simulink model "FCS"  (R2019a)
settings: Solver=VariableStepAuto  StartTime=0.0  StopTime=10.0  RelTol=1e-3
undefined symbols (not defined in the file): argentina, ground, JD_0, Jw, namibia, nut80, r_ecef, t_orbit, v_ecef
libraries: dspmathops x12, vrlib x8, sc_toolbox x7
(part 1 of 2)
settings Model: Creator=mario  LastModifiedBy=mario
settings DataIOCC: ReturnWorkspaceOutputs=off
settings DebuggingCC: ArithmeticOperatorsInVariantConditions=warning
settings ModelReferenceCC: ModelReferenceNumInstancesAllowed=Single

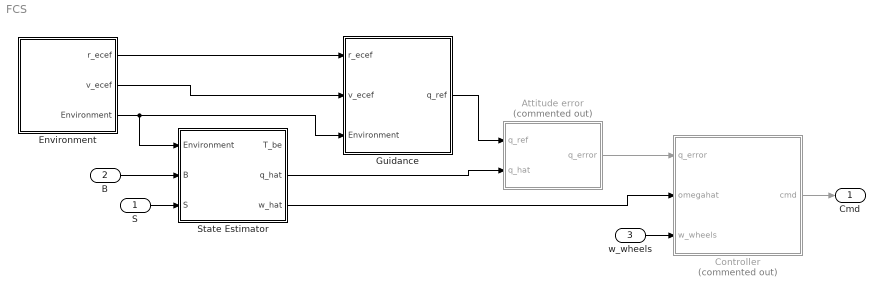
== system FCS ==
  S : Inport
  B : Inport  Port=2
  w_wheels : Inport  Port=3
  Attitude error : Subsystem  Commented=on
  Controller : Subsystem  Commented=on
  Environment : Subsystem
  Guidance : Subsystem
  State Estimator : Subsystem
  Cmd : Outport
  wires:
  Attitude error/1("q_error ") -> Controller/1(q_error)
  Controller/1(cmd) -> Cmd/1
  State Estimator/2(q_hat) -> Attitude error/2(q_hat)
  Guidance/1(q_ref) -> Attitude error/1(q_ref)
  w_wheels/1 -> Controller/3(w_wheels)
  State Estimator/3(w_hat) -> Controller/2(omegahat)
  B/1 -> State Estimator/2(B)
  S/1 -> State Estimator/3(S)
  Environment/1(r_ecef) -> Guidance/1(r_ecef)
  Environment/2(v_ecef) -> Guidance/2(v_ecef)
  Environment/3(Environment) -> State Estimator/1("Environment "), Guidance/3(Environment)

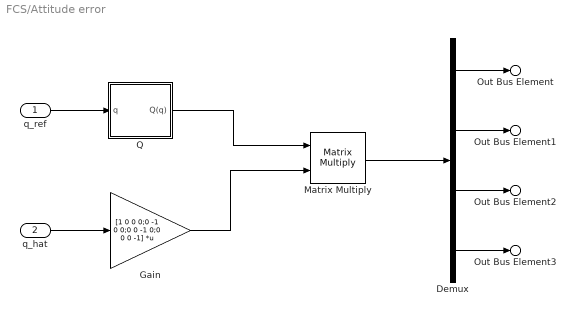
== system FCS/Attitude error ==
  q_ref : Inport
  q_hat : Inport  Port=2
  Demux : Demux
  Gain : Gain  Gain=[1 0 0 0;0 -1 0 0;0 0 -1 0;0 0 0 -1]  Multiplication=Matrix(K*u)
  Matrix Multiply : Product  Multiplication=Matrix(*)
  Q : Subsystem
  Out Bus Element : Outport  PortName=q_error  Element=q0
  Out Bus Element1 : Outport  PortName=q_error  Element=q1
  Out Bus Element2 : Outport  PortName=q_error  Element=q2
  Out Bus Element3 : Outport  PortName=q_error  Element=q3
  wires:
  q_ref/1 -> Q/1(q)
  q_hat/1 -> Gain/1
  Q/1(Q(q)) -> Matrix Multiply/1
  Gain/1 -> Matrix Multiply/2
  Matrix Multiply/1 -> Demux/1
  Demux/1 -> Out Bus Element/1
  Demux/3 -> Out Bus Element2/1
  Demux/2 -> Out Bus Element1/1
  Demux/4 -> Out Bus Element3/1

== system FCS/Controller ==
  q_error : Inport
  omegahat : Inport  Port=2
  w_wheels : Inport  Port=3
  Detumbling : Subsystem
  Momemtum unloading : Subsystem
  Three axis attitude controller : Subsystem
  cmd : Outport
  wires:
  Three axis attitude controller/1("cmd ") -> cmd/1
  q_error/1 -> Three axis attitude controller/1(q_error)
  omegahat/1 -> Three axis attitude controller/2(w_body)
  w_wheels/1 -> Momemtum unloading/1(w_wheels)

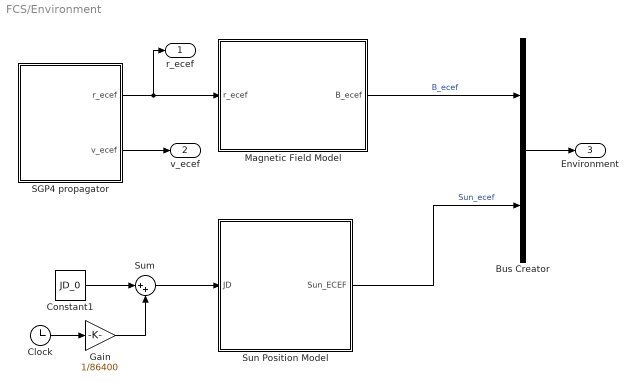
== system FCS/Environment ==
  Bus Creator : BusCreator  Inputs=2
  Clock : Clock
  Constant1 : Constant  Value=JD_0
  Gain : Gain  Gain=1/86400
  Magnetic Field Model : Subsystem
  SGP4 propagator : Subsystem
  Sum : Sum  Inputs=|++
  "Sun Position Model " : Subsystem
  r_ecef : Outport
  v_ecef : Outport  Port=2
  Environment : Outport  Port=3
  wires:
  Clock/1 -> Gain/1
  Constant1/1 -> Sum/1
  Gain/1 -> Sum/2
  Sum/1 -> "Sun Position Model "/1(JD)
  Magnetic Field Model/1(B_ecef) -> Bus Creator/1  "B_ecef"
  "Sun Position Model "/1(Sun_ECEF) -> Bus Creator/2  "Sun_ecef"
  Bus Creator/1 -> Environment/1
  SGP4 propagator/1(r_ecef) -> r_ecef/1, Magnetic Field Model/1(r_ecef)
  SGP4 propagator/2(v_ecef) -> v_ecef/1

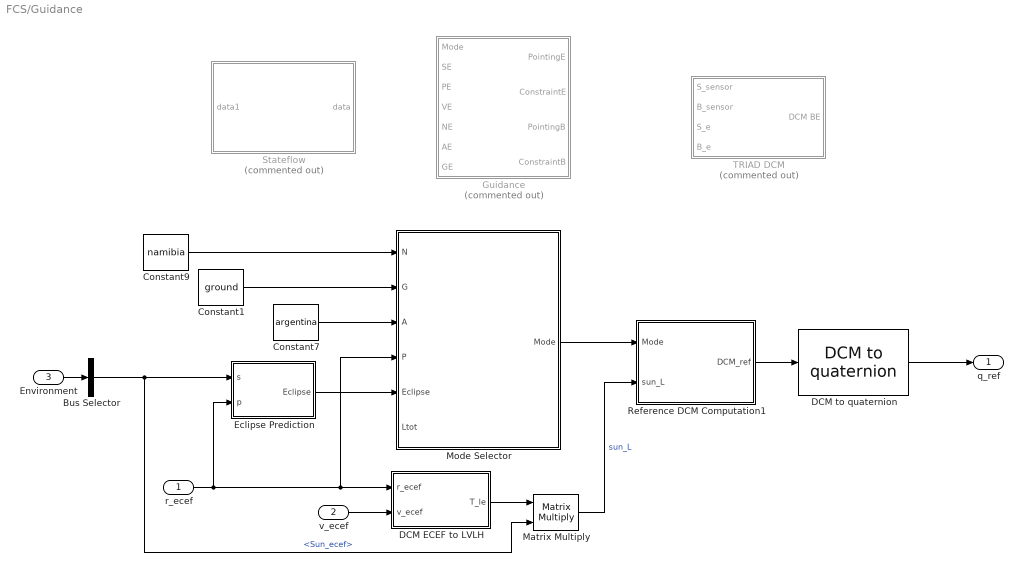
== system FCS/Guidance ==
  r_ecef : Inport
  v_ecef : Inport  Port=2
  Environment : Inport  Port=3
  Bus Selector : BusSelector  OutputSignals=Sun_ecef
  Constant1 : Constant  Value=ground
  Constant7 : Constant  Value=argentina
  Constant9 : Constant  Value=namibia
  DCM ECEF to LVLH : Subsystem
  DCM to quaternion : sc_toolbox/Kinematics/DCM to quaternion  SystemSampleTime=-1
      settings: SourceProductName=Spacecraft Toolbox
  Eclipse Prediction : MATLAB Function  TreatAsAtomicUnit=on
  Guidance : MATLAB Function  Commented=on  TreatAsAtomicUnit=on
  Matrix Multiply : Product  Multiplication=Matrix(*)
  Mode Selector : MATLAB Function  TreatAsAtomicUnit=on
  Reference DCM Computation1 : MATLAB Function  TreatAsAtomicUnit=on
  Stateflow : Stateflow chart  Commented=on  TreatAsAtomicUnit=on
  TRIAD DCM : Subsystem  Commented=on
  q_ref : Outport  VectorParamsAs1DForOutWhenUnconnected=on
  wires:
  Constant1/1 -> Mode Selector/2(G)
  Constant9/1 -> Mode Selector/1(N)
  Constant7/1 -> Mode Selector/3(A)
  Eclipse Prediction/1(Eclipse) -> Mode Selector/5(Eclipse)
  Mode Selector/1(Mode) -> Reference DCM Computation1/1(Mode)
  v_ecef/1 -> DCM ECEF to LVLH/2(v_ecef)
  DCM to quaternion/1 -> q_ref/1
  Reference DCM Computation1/1(DCM_ref) -> DCM to quaternion/1
  r_ecef/1 -> Eclipse Prediction/2(p), DCM ECEF to LVLH/1(r_ecef), Mode Selector/4(P)
  Environment/1 -> Bus Selector/1
  Bus Selector/1 -> Matrix Multiply/2, Eclipse Prediction/1(s)  "<Sun_ecef>"
  DCM ECEF to LVLH/1(T_le) -> Matrix Multiply/1
  Matrix Multiply/1 -> Reference DCM Computation1/2(sun_L)  "sun_L"

== system FCS/State Estimator ==
  "Environment " : Inport
  B : Inport  Port=2
  S : Inport  Port=3
  Bus Selector : BusSelector  OutputSignals=B_ecef,Sun_ecef
  Extended Kalman Filter : MATLAB Function  Commented=on  TreatAsAtomicUnit=on
  TRIAD DCM : Subsystem
  T_be : Outport
  q_hat : Outport  Port=2
  w_hat : Outport  Port=3
  wires:
  B/1 -> TRIAD DCM/2(B_sensor), Extended Kalman Filter/1(B)
  S/1 -> TRIAD DCM/1(S_sensor), Extended Kalman Filter/2(S)
  Extended Kalman Filter/2(what) -> w_hat/1
  Extended Kalman Filter/1(qhat) -> q_hat/1
  TRIAD DCM/1(DCM BE) -> T_be/1
  "Environment "/1 -> Bus Selector/1
  Bus Selector/1 -> TRIAD DCM/3(B_e)  "<B_ecef>"
  Bus Selector/2 -> TRIAD DCM/4(S_e)  "<Sun_ecef>"

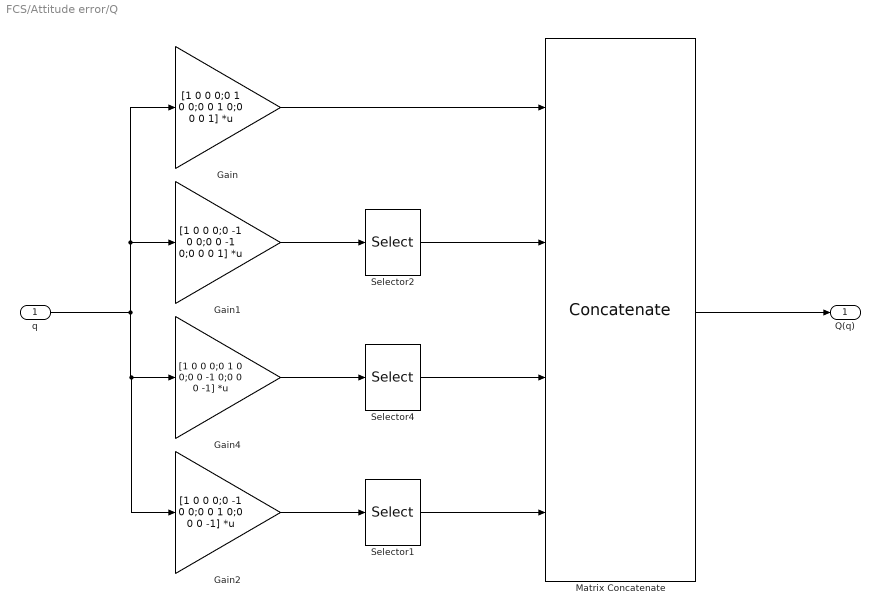
== system FCS/Attitude error/Q ==
  q : Inport
  Gain : Gain  Gain=[1 0 0 0;0 1 0 0;0 0 1 0;0 0 0 1]  Multiplication=Matrix(K*u)
  Gain1 : Gain  Gain=[1 0 0 0;0 -1 0 0;0 0 -1 0;0 0 0 1]  Multiplication=Matrix(K*u)
  Gain2 : Gain  Gain=[1 0 0 0;0 -1 0 0;0 0 1 0;0 0 0 -1]  Multiplication=Matrix(K*u)
  Gain4 : Gain  Gain=[1 0 0 0;0 1 0 0;0 0 -1 0;0 0 0 -1]  Multiplication=Matrix(K*u)
  Matrix Concatenate : Concatenate  NumInputs=4  Mode=Multidimensional array  ConcatenateDimension=2
  Selector1 : Selector  InputPortWidth=4  IndexOptions=Index vector (dialog)  Indices=[4 3 2 1]  OutputSizes=1
  Selector2 : Selector  InputPortWidth=4  IndexOptions=Index vector (dialog)  Indices=[2 1 4 3]  OutputSizes=1
  Selector4 : Selector  InputPortWidth=4  IndexOptions=Index vector (dialog)  Indices=[3 4 1 2]  OutputSizes=1
  Q(q) : Outport
  wires:
  Gain1/1 -> Selector2/1
  Gain/1 -> Matrix Concatenate/1
  q/1 -> Gain2/1, Gain4/1, Gain1/1, Gain/1
  Selector4/1 -> Matrix Concatenate/3
  Matrix Concatenate/1 -> Q(q)/1
  Selector2/1 -> Matrix Concatenate/2
  Gain4/1 -> Selector4/1
  Gain2/1 -> Selector1/1
  Selector1/1 -> Matrix Concatenate/4

== system FCS/Controller/Detumbling ==
  In1 : Inport
  cmd : Outport
  wires:
  In1/1 -> cmd/1

== system FCS/Controller/Momemtum unloading ==
  w_wheels : Inport
  cmd : Outport
  wires:
  w_wheels/1 -> cmd/1

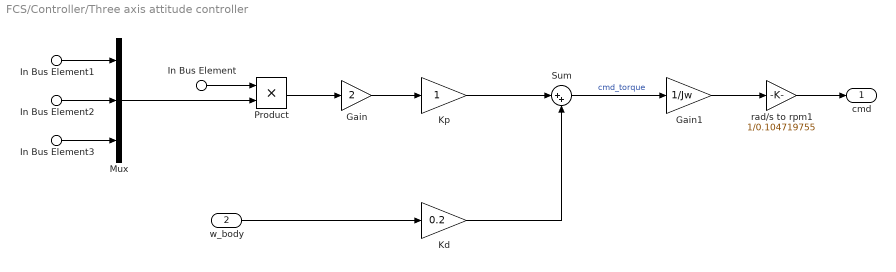
== system FCS/Controller/Three axis attitude controller ==
  In Bus Element : Inport  PortName=q_error  Element=q0
  In Bus Element1 : Inport  PortName=q_error  Element=q1
  In Bus Element2 : Inport  PortName=q_error  Element=q2
  In Bus Element3 : Inport  PortName=q_error  Element=q3
  w_body : Inport  Port=2
  Gain : Gain  Gain=2
  Gain1 : Gain  Gain=1/Jw
  Kd : Gain  Gain=0.2
  Kp : Gain
  Mux : Mux  Inputs=3
  Product : Product
  Sum : Sum  Inputs=|++
  rad/s to rpm1 : Gain  Gain=1/0.104719755
  "cmd " : Outport
  wires:
  w_body/1 -> Kd/1
  In Bus Element1/1 -> Mux/1
  Gain1/1 -> rad/s to rpm1/1
  Mux/1 -> Product/2
  Gain/1 -> Kp/1
  Product/1 -> Gain/1
  Kd/1 -> Sum/2
  In Bus Element2/1 -> Mux/2
  rad/s to rpm1/1 -> "cmd "/1
  In Bus Element/1 -> Product/1
  In Bus Element3/1 -> Mux/3
  Sum/1 -> Gain1/1  "cmd_torque"
  Kp/1 -> Sum/1

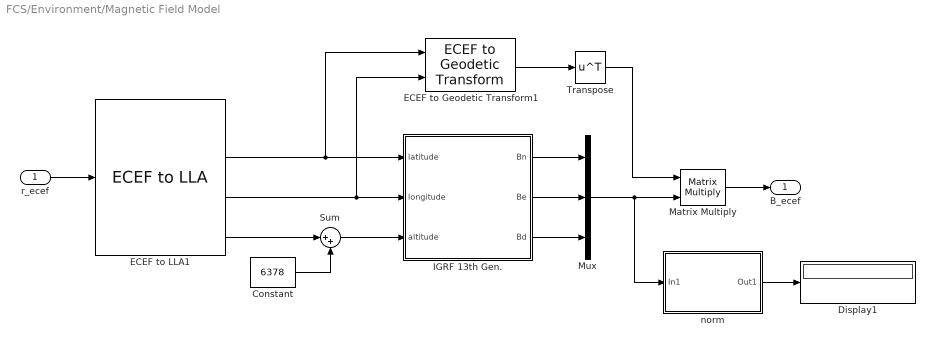
== system FCS/Environment/Magnetic Field Model ==
  r_ecef : Inport
  Constant : Constant  Value=6378
  Display1 : Display
  ECEF to Geodetic Transform1 : sc_toolbox/Coordinates Transformations/ECEF to Geodetic Transform  SystemSampleTime=-1
      settings: SourceProductName=Spacecraft Toolbox
  ECEF to LLA1 : sc_toolbox/Coordinates Transformations/ECEF to LLA  SystemSampleTime=-1
      settings: SourceProductName=Spacecraft Toolbox
  IGRF 13th Gen. : MATLAB Function  TreatAsAtomicUnit=on
  Matrix Multiply : Product  Multiplication=Matrix(*)
  Mux : Mux  Inputs=3
  Sum : Sum  Inputs=|++
  Transpose : Math  Operator=transpose  SaturateOnIntegerOverflow=on
  norm : Subsystem
  B_ecef : Outport  VectorParamsAs1DForOutWhenUnconnected=on
  wires:
  IGRF 13th Gen./2(Be) -> Mux/2
  IGRF 13th Gen./3(Bd) -> Mux/3
  IGRF 13th Gen./1(Bn) -> Mux/1
  r_ecef/1 -> ECEF to LLA1/1
  ECEF to LLA1/3 -> ECEF to Geodetic Transform1/2, IGRF 13th Gen./2(longitude)
  ECEF to LLA1/2 -> ECEF to Geodetic Transform1/1, IGRF 13th Gen./1(latitude)
  ECEF to LLA1/4 -> Sum/1
  Mux/1 -> Matrix Multiply/2, norm/1(In1)
  Sum/1 -> IGRF 13th Gen./3(altitude)
  Constant/1 -> Sum/2
  norm/1(Out1) -> Display1/1
  ECEF to Geodetic Transform1/1 -> Transpose/1
  Matrix Multiply/1 -> B_ecef/1
  Transpose/1 -> Matrix Multiply/1

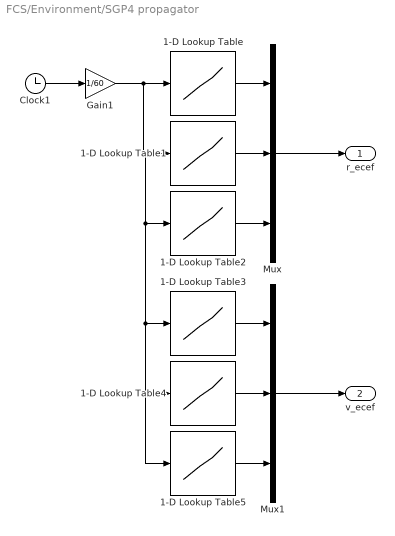
== system FCS/Environment/SGP4 propagator ==
  1-D Lookup Table : Lookup_n-D  NumberOfTableDimensions=1  BreakpointsForDimension1=t_orbit  BreakpointsForDimension2=t_orbit  BreakpointsForDimension3=t_orbit  Table=r_ecef(:,1)  InternalRulePriority=Speed  RndMeth=Simplest  InputSameDT=on
  1-D Lookup Table1 : Lookup_n-D  NumberOfTableDimensions=1  BreakpointsForDimension1=t_orbit  BreakpointsForDimension2=t_orbit  BreakpointsForDimension3=t_orbit  Table=r_ecef(:,2)  InternalRulePriority=Speed  RndMeth=Simplest  InputSameDT=on
  1-D Lookup Table2 : Lookup_n-D  NumberOfTableDimensions=1  BreakpointsForDimension1=t_orbit  BreakpointsForDimension2=t_orbit  BreakpointsForDimension3=t_orbit  Table=r_ecef(:,3)  InternalRulePriority=Speed  RndMeth=Simplest  InputSameDT=on
  1-D Lookup Table3 : Lookup_n-D  NumberOfTableDimensions=1  BreakpointsForDimension1=t_orbit  BreakpointsForDimension2=t_orbit  BreakpointsForDimension3=t_orbit  Table=v_ecef(:,1)  InternalRulePriority=Speed  RndMeth=Simplest  InputSameDT=on
  1-D Lookup Table4 : Lookup_n-D  NumberOfTableDimensions=1  BreakpointsForDimension1=t_orbit  BreakpointsForDimension2=t_orbit  BreakpointsForDimension3=t_orbit  Table=v_ecef(:,2)  InternalRulePriority=Speed  RndMeth=Simplest  InputSameDT=on
  1-D Lookup Table5 : Lookup_n-D  NumberOfTableDimensions=1  BreakpointsForDimension1=t_orbit  BreakpointsForDimension2=t_orbit  BreakpointsForDimension3=t_orbit  Table=v_ecef(:,3)  InternalRulePriority=Speed  RndMeth=Simplest  InputSameDT=on
  Clock1 : Clock
  Gain1 : Gain  Gain=1/60
  Mux : Mux  Inputs=3
  Mux1 : Mux  Inputs=3
  r_ecef : Outport  VectorParamsAs1DForOutWhenUnconnected=on
  v_ecef : Outport  Port=2
  wires:
  1-D Lookup Table2/1 -> Mux/3
  Gain1/1 -> 1-D Lookup Table5/1, 1-D Lookup Table4/1, 1-D Lookup Table3/1, 1-D Lookup Table2/1, 1-D Lookup Table1/1, 1-D Lookup Table/1
  Clock1/1 -> Gain1/1
  1-D Lookup Table1/1 -> Mux/2
  1-D Lookup Table/1 -> Mux/1
  Mux/1 -> r_ecef/1
  1-D Lookup Table3/1 -> Mux1/1
  1-D Lookup Table4/1 -> Mux1/2
  1-D Lookup Table5/1 -> Mux1/3
  Mux1/1 -> v_ecef/1

== system FCS/Environment/Sun Position Model  ==
  JD : Inport
  MOD to ECEF : Subsystem
  Sun Position Vector : MATLAB Function  TreatAsAtomicUnit=on
  Sun_ECEF : Outport
  wires:
  Sun Position Vector/1(rsun) -> MOD to ECEF/1(Sun_MOD)
  JD/1 -> MOD to ECEF/2(JD), Sun Position Vector/1(jd)
  MOD to ECEF/1(Sun_ECEF) -> Sun_ECEF/1

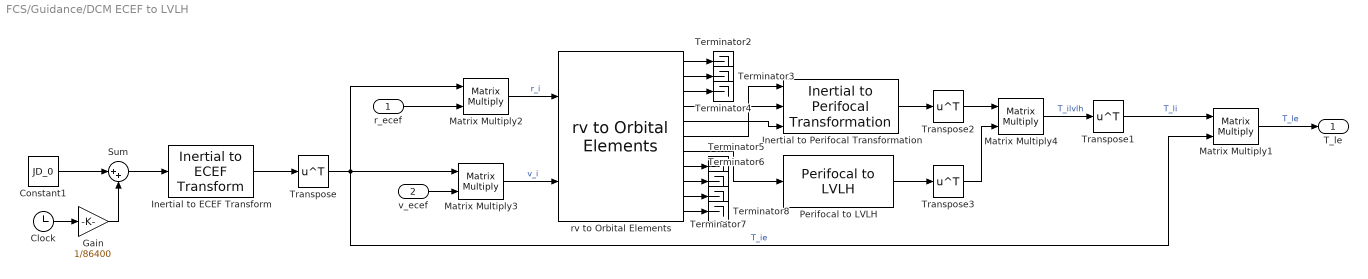
== system FCS/Guidance/DCM ECEF to LVLH ==
  r_ecef : Inport
  v_ecef : Inport  Port=2
  Clock : Clock
  Constant1 : Constant  Value=JD_0
  Gain : Gain  Gain=1/86400
  Inertial to ECEF Transform : sc_toolbox/Inertial to ECEF Transform  SystemSampleTime=-1
      settings: SourceProductName=Spacecraft Toolbox
  Inertial to Perifocal Transformation : sc_toolbox/Inertial to Perifocal Transformation  SystemSampleTime=-1
      settings: SourceProductName=Spacecraft Toolbox
  Matrix Multiply{1..4} (4 alike) : Product  Multiplication=Matrix(*)
  Perifocal to LVLH : sc_toolbox/Perifocal to LVLH  SystemSampleTime=-1
      settings: SourceProductName=Spacecraft Toolbox
  Sum : Sum  Inputs=|++
  Terminator{2..8} (7 alike) : Terminator
  Transpose{,1..3} (4 alike) : Math  Operator=transpose  SaturateOnIntegerOverflow=on
  rv to Orbital Elements : sc_toolbox/rv to Orbital Elements  SystemSampleTime=-1
      settings: SourceProductName=Spacecraft Toolbox
  T_le : Outport
  wires:
  rv to Orbital Elements/7 -> Perifocal to LVLH/1
  Matrix Multiply4/1 -> Transpose1/1  "T_ilvlh"
  Transpose3/1 -> Matrix Multiply4/2
  Matrix Multiply2/1 -> rv to Orbital Elements/1  "r_i"
  rv to Orbital Elements/2 -> Terminator3/1
  Perifocal to LVLH/1 -> Transpose3/1
  Transpose2/1 -> Matrix Multiply4/1
  rv to Orbital Elements/1 -> Terminator2/1
  rv to Orbital Elements/8 -> Terminator5/1
  rv to Orbital Elements/3 -> Terminator4/1
  Inertial to Perifocal Transformation/1 -> Transpose2/1
  rv to Orbital Elements/6 -> Inertial to Perifocal Transformation/1
  rv to Orbital Elements/11 -> Terminator8/1
  Matrix Multiply3/1 -> rv to Orbital Elements/2  "v_i"
  rv to Orbital Elements/5 -> Inertial to Perifocal Transformation/3
  rv to Orbital Elements/10 -> Terminator7/1
  rv to Orbital Elements/9 -> Terminator6/1
  rv to Orbital Elements/4 -> Inertial to Perifocal Transformation/2
  v_ecef/1 -> Matrix Multiply3/2
  Sum/1 -> Inertial to ECEF Transform/1
  Inertial to ECEF Transform/1 -> Transpose/1
  Constant1/1 -> Sum/1
  Gain/1 -> Sum/2
  Clock/1 -> Gain/1
  r_ecef/1 -> Matrix Multiply2/2
  Matrix Multiply1/1 -> T_le/1  "T_le"
  Transpose1/1 -> Matrix Multiply1/1  "T_li"
  Transpose/1 -> Matrix Multiply1/2, Matrix Multiply2/1, Matrix Multiply3/1  "T_ie"

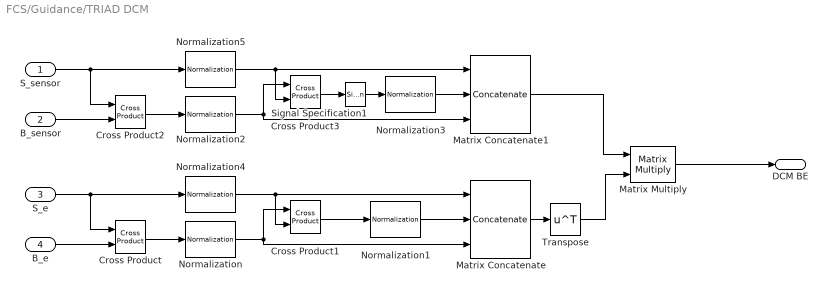
== system FCS/Guidance/TRIAD DCM ==
  S_sensor : Inport
  B_sensor : Inport  Port=2
  S_e : Inport  Port=3
  B_e : Inport  Port=4
  Cross Product{,1..3} (4 alike) : vrlib/Utilities/Cross Product
      settings: SourceProductBaseCode=VR
  Matrix Concatenate : Concatenate  NumInputs=3  Mode=Multidimensional array  ConcatenateDimension=2
  Matrix Concatenate1 : Concatenate  NumInputs=3  Mode=Multidimensional array  ConcatenateDimension=2
  Matrix Multiply : Product  Multiplication=Matrix(*)
  Normalization{,1..5} (6 alike) : dspmathops/Normalization  NormType=2-norm  Bias=1e-10  NormOver=Each column  Dimension=1  roundingMode=Floor  overflowMode=off  accumDataTypeStr=Inherit: Same as product output  accumLastDataTypeStr=Inherit: Same as product output  outputDataTypeStr=Inherit: Same as product output  outputMin=[]  outputMax=[]  outputLastDataTypeStr=Inherit: Same as product output
      settings: SourceProductName=DSP System Toolbox
  Signal Specification1 : SignalSpecification  Dimensions=3
  Transpose : Math  Operator=transpose  SaturateOnIntegerOverflow=on
  DCM BE : Outport
  wires:
  Normalization/1 -> Matrix Concatenate/3, Cross Product1/1
  Normalization5/1 -> Matrix Concatenate1/1, Cross Product3/2
  Cross Product1/1 -> Normalization1/1
  Normalization3/1 -> Matrix Concatenate1/2
  Cross Product3/1 -> Signal Specification1/1
  B_e/1 -> Cross Product/2
  Normalization4/1 -> Matrix Concatenate/1, Cross Product1/2
  S_e/1 -> Normalization4/1, Cross Product/1
  Cross Product2/1 -> Normalization2/1
  Cross Product/1 -> Normalization/1
  Normalization1/1 -> Matrix Concatenate/2
  Normalization2/1 -> Cross Product3/1, Matrix Concatenate1/3
  Matrix Concatenate/1 -> Transpose/1
  Matrix Concatenate1/1 -> Matrix Multiply/1
  Transpose/1 -> Matrix Multiply/2
  S_sensor/1 -> Cross Product2/1, Normalization5/1
  B_sensor/1 -> Cross Product2/2
  Matrix Multiply/1 -> DCM BE/1
  Signal Specification1/1 -> Normalization3/1

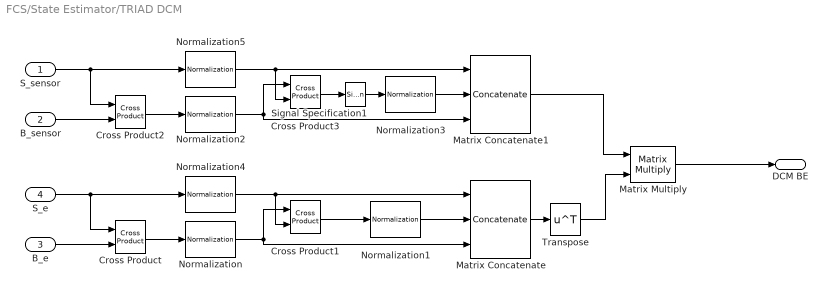
== system FCS/State Estimator/TRIAD DCM ==
  S_sensor : Inport
  B_sensor : Inport  Port=2
  B_e : Inport  Port=3
  S_e : Inport  Port=4
  Cross Product{,1..3} (4 alike) : vrlib/Utilities/Cross Product
      settings: SourceProductBaseCode=VR
  Matrix Concatenate : Concatenate  NumInputs=3  Mode=Multidimensional array  ConcatenateDimension=2
  Matrix Concatenate1 : Concatenate  NumInputs=3  Mode=Multidimensional array  ConcatenateDimension=2
  Matrix Multiply : Product  Multiplication=Matrix(*)
  Normalization{,1..5} (6 alike) : dspmathops/Normalization  NormType=2-norm  Bias=1e-10  NormOver=Each column  Dimension=1  roundingMode=Floor  overflowMode=off  accumDataTypeStr=Inherit: Same as product output  accumLastDataTypeStr=Inherit: Same as product output  outputDataTypeStr=Inherit: Same as product output  outputMin=[]  outputMax=[]  outputLastDataTypeStr=Inherit: Same as product output
      settings: SourceProductName=DSP System Toolbox
  Signal Specification1 : SignalSpecification  Dimensions=3
  Transpose : Math  Operator=transpose  SaturateOnIntegerOverflow=on
  DCM BE : Outport
  wires:
  Normalization/1 -> Matrix Concatenate/3, Cross Product1/1
  Normalization5/1 -> Matrix Concatenate1/1, Cross Product3/2
  Cross Product1/1 -> Normalization1/1
  Normalization3/1 -> Matrix Concatenate1/2
  Cross Product3/1 -> Signal Specification1/1
  B_e/1 -> Cross Product/2
  Normalization4/1 -> Matrix Concatenate/1, Cross Product1/2
  S_e/1 -> Normalization4/1, Cross Product/1
  Cross Product2/1 -> Normalization2/1
  Cross Product/1 -> Normalization/1
  Normalization1/1 -> Matrix Concatenate/2
  Normalization2/1 -> Cross Product3/1, Matrix Concatenate1/3
  Matrix Concatenate/1 -> Transpose/1
  Matrix Concatenate1/1 -> Matrix Multiply/1
  Transpose/1 -> Matrix Multiply/2
  S_sensor/1 -> Cross Product2/1, Normalization5/1
  B_sensor/1 -> Cross Product2/2
  Matrix Multiply/1 -> DCM BE/1
  Signal Specification1/1 -> Normalization3/1

== system FCS/Environment/Magnetic Field Model/norm ==
  In1 : Inport
  Add : Sum  Inputs=+++
  Demux : Demux  Outputs=3
  Product : Product
  Product1 : Product
  Product2 : Product
  Sqrt : Sqrt  SaturateOnIntegerOverflow=on
  Out1 : Outport
  wires:
  Demux/2 -> Product1/2, Product1/1
  Demux/1 -> Product/2, Product/1
  Sqrt/1 -> Out1/1
  Product2/1 -> Add/3
  Product1/1 -> Add/2
  Product/1 -> Add/1
  Add/1 -> Sqrt/1
  Demux/3 -> Product2/2, Product2/1
  In1/1 -> Demux/1

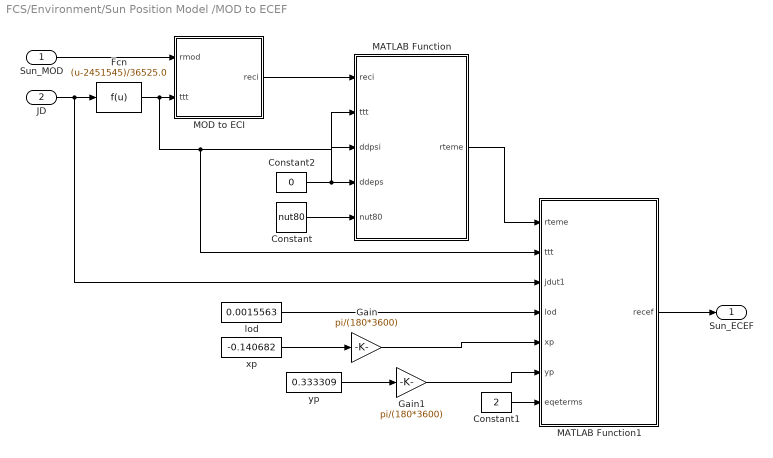
== system FCS/Environment/Sun Position Model /MOD to ECEF ==
  Sun_MOD : Inport
  JD : Inport  Port=2
  Constant : Constant  Value=nut80
  Constant1 : Constant  Value=2
  Constant2 : Constant  Value=0
  Fcn : Fcn  Expr=(u-2451545)/36525.0
  Gain : Gain  Gain=pi/(180*3600)
  Gain1 : Gain  Gain=pi/(180*3600)
  MATLAB Function : MATLAB Function  TreatAsAtomicUnit=on
  MATLAB Function1 : MATLAB Function  TreatAsAtomicUnit=on
  MOD to ECI : MATLAB Function  TreatAsAtomicUnit=on
  lod : Constant  Value=0.0015563
  xp : Constant  Value=-0.140682
  yp : Constant  Value=0.333309
  Sun_ECEF : Outport
  wires:
  Sun_MOD/1 -> MOD to ECI/1(rmod)
  Fcn/1 -> MATLAB Function1/2(ttt), MATLAB Function/2(ttt), MOD to ECI/2(ttt)
  JD/1 -> MATLAB Function1/3(jdut1), Fcn/1
  MOD to ECI/1(reci) -> MATLAB Function/1(reci)
  Constant2/1 -> MATLAB Function/4(ddeps), MATLAB Function/3(ddpsi)
  MATLAB Function1/1(recef) -> Sun_ECEF/1
  MATLAB Function/1(rteme) -> MATLAB Function1/1(rteme)
  Constant/1 -> MATLAB Function/5(nut80)
  Constant1/1 -> MATLAB Function1/7(eqeterms)
  lod/1 -> MATLAB Function1/4(lod)
  Gain/1 -> MATLAB Function1/5(xp)
  yp/1 -> Gain1/1
  xp/1 -> Gain/1
  Gain1/1 -> MATLAB Function1/6(yp)

== matlab function FCS/State Estimator/Extended Kalman Filter ==
  data: B input; qhat output; S input; what output
function [qhat,what] = ekf(B,S)
% QUATERNIONS EKF

% Initialization
T = 1/30;
g = 9.81;
n = length(acc);
euler = zeros(n,3);
euler(1,:) = [0 0 0];

x_hatp = [euler3212q(euler(1,:));zeros(3,1)];
Pp = 0.0001*eye(7);
R =diag([8e-4;8e-4;8e-4]);
qq = 0.0001;
qb = 1e-5;
Q =diag([qq;qq;qq;qq;qb;qb;qb]);

for i = 1:n
    
    Sq = [-x_hatp(2) -x_hatp(3) -x_hatp(4);
    x_hatp(1) -x_hatp(4) x_hatp(3);
    x_hatp(4) x_hatp(1) -x_hatp(2);
    -x_hatp(3) x_hatp(2) x_hatp(1)];

    Sw = [0 -gyr(i,1) -gyr(i,2) -gyr(i,3);
        gyr(i,1) 0 gyr(i,3) -gyr(i,2);
        gyr(i,2) -gyr(i,3) 0 gyr(i,1);
        gyr(i,3) gyr(i,2) -gyr(i,1) 0]; 
    
    F = [0.5*Sw -0.5*Sq;
        zeros(3,4) zeros(3,3)];
    
    Phi = expm(F*T);
    func = @(x)Phi*Q*Phi';
    Q_m = integral(func,0,T,'ArrayValued',1,'RelTol',5);
    
    Qk = [T^3/12*(qq*(eye(4)+Sw)*(eye(4)+Sw'))+qb*Sq*(Sq') -T^2/4*qb*Sq;
        -T^2/4*qb*Sq' T*qb*eye(3)];
    
    % Propagation

    x_hatm = Phi*x_hatp;
    Pm = Phi*Pp*Phi' + Q_m;
    %x_hatm(1:4) = x_hatm(1:4)/norm(x_hatm(1:4));
    
    % Measurement

    H =  2*[-x_hatm(3) x_hatm(4) -x_hatm(1) x_hatm(2) zeros(1,3);
                x_hatm(2) x_hatm(1) x_hatm(4) x_hatm(3) zeros(1,3);
                x_hatm(1) -x_hatm(2) -x_hatm(3) x_hatm(4) zeros(1,3)];

    y_hat = H*x_hatm;
    S = (H*Pm*H'+R);
    K = (H*Pm)'/S;

    % Update
    y = [acc(i,1)/g acc(i,2)/g acc(i,3)/g]';
    x_hatp = x_hatm + K*(y - y_hat);
    Pp = (eye(7) - K*H)*Pm;
    
    x_hatp(1:4) = x_hatp(1:4)/norm(x_hatp(1:4));
    euler(i,:) = q2euler(x_hatp(1:4));
    
end

== stateflow chart FCS/Guidance/Stateflow ==
  state Mission_modes
    state Idle
    state Imaging
    (default) -> Idle
  (default) -> Mission_modes
  data: data output; data1 input

== matlab function FCS/Environment/Magnetic Field Model/IGRF 13th Gen. ==
  data: latitude input; Bn output; longitude input; altitude input; Be output; Bd output
function [Bn, Be, Bd] = igrf(latitude, longitude, altitude)

%REMOVED COORD AS EVERYTHING IS ALREADY IN GEOCENTRIC. KEEPING TIME FOR NOW

% IGRF Earth's magnetic field from IGRF model.
% 
% Usage: [BX, BY, BZ] = IGRF(TIME, LATITUDE, LONGITUDE, ALTITUDE, COORD)
%     or [BX, BY, BZ] = IGRF(COEFS, LATITUDE, LONGITUDE, ALTITUDE, COORD)
%     or B = IGRF(TIME, LATITUDE, LONGITUDE, ALTITUDE, COORD)
%     or B = IGRF(COEFS, LATITUDE, LONGITUDE, ALTITUDE, COORD)
% 
% Calculates the components of the Earth's magnetic field using the
% International Geomagnetic Reference Field (IGRF) model. The inputs for
% the position can be scalars or vectors (in the latter case each should
% have the same number of elements or be a scalar), but TIME must be a
% scalar.
% 
% When all the coordinate inputs are scalars, the function can be run more
% efficiently by providing the proper IGRF coefficient vector for a given
% time rather than the time itself. This mode is useful when making
% multiple calls to the function while keeping the time the same (meaning
% the coefficients will be the same for each run) as loading the
% coefficients can be the most time-consuming part of the function. The
% coefficient vector can be easily loaded using the function LOADIGRFCOEFS.
% This mode is assumed when all the coordinate inputs are scalars and the
% first input is a vector. In this case, the coefficient vector should be
% formatted as (LOADIGRFCOEFS provides this):
% 
%   [g(n=1,m=0) g(n=1,m=1) h(n=1,m=1) g(n=2,m=0) g(n=2,m=1) h(n=2,m=1) ...]
% 
% Regardless of the size of the inputs, the outputs will be column vectors.
% If only one output is requested, B = [BX(:), BY(:), BZ(:)] is output.
% Note that the other parameters the IGRF gives can be computed from BX,
% BY, and BZ as:
% 
%   Horizonal intensity: hypot(BX, BY) (i.e., sqrt(BX.^2 + BY.^2) )
%   Total intensity: hypot(BX, hypot(BY, BZ))
%   Declination: atan2(BY, BX)
%   Inclination: atan(BZ./hypot(BX, BY))
% 
% This function relies on having the file igrfcoefs.mat in the MATLAB
% path to function properly when a time is input. If this file cannot be
% found, this function will try to create it by calling GETIGRFCOEFS.
% 
% The IGRF is a spherical harmonic expansion of the Earth's internal
% magnetic field. Currently, the IGRF model is valid between the years 1900
% and 2015. See the health warning for the IGRF model here:
% http://www.ngdc.noaa.gov/IAGA/vmod/igrfhw.html
% 
% Reference:
% International Association of Geomagnetism and Aeronomy, Working Group 
% V-MOD (2010), International Geomagnetic Reference Field: the eleventh
% generation, _Geophys. J. Int._, _183_(3), 1216-1230, 
% doi:10.1111/j.1365-246X.2010.04804.x.
% 
% Inputs:
%   -TIME: Time to get the magnetic field values either in MATLAB serial
%   date number format or a string that can be converted into MATLAB serial
%   date number format using DATENUM with no format specified (see
%   documentation of DATENUM for more information).
%   -COEFS: Instead of inputting a time, you can simply specify the proper
%   coefficients for the time you want by inputting in the first argument
%   the proper coefficient vector from igrfcoefs.mat.
%   -LATITUDE: Geocentric or geodetic latitude in degrees. **SCODIN**In radian
%   -LONGITUDE: Geocentric or geodetic longitude in degrees. **SCODIN**In radian
%   -ALTITUDE: For geodetic coordiates, the height in km above the Earth's
%   surface. For geocentric coordiates, the radius in km from the center of
%   the Earth.
%   -COORD: String specifying the coordinate system to use. Either
%   'geocentric' or 'geodetic' (optional, default is geodetic). Note that
%   only geodetic coordinates have been verified.
% 
% Outputs:
%   -BX: Northward component of the magnetic field in nanoteslas (nT).
%   -BY: Eastward component of the magnetic field in nT.
%   -BZ: Downward component of the magnetic field in nT.
%   -B: [BX(:), BY(:), BZ(:)].
% 
% See also: LOADIGRFCOEFS, GETIGRFCOEFS, IGRFLINE, DATENUM, IGRF11MAGM.

% Run IGRFS if all position inputs are scalars.
if isscalar(latitude) && isscalar(longitude) && isscalar(altitude)
        [Bn, Be, Bd] = igrfs(latitude, longitude, altitude);
end

if nargout <= 1
    Bn = [Bn(:), Be(:), Bd(:)];
end
%%%%%%%%%%%%%%%%%%%%%%%%%%%%%%%%%%%%%%%%%%%%%%%%%%%%%%%%%%%%%%%%%%%%%%%%%%%
%%%%%%%%%%%%%%%%%%%        IGRF scalar function.        %%%%%%%%%%%%%%%%%%%
%%%%%%%%%%%%%%%%%%%%%%%%%%%%%%%%%%%%%%%%%%%%%%%%%%%%%%%%%%%%%%%%%%%%%%%%%%%
function [Bn, Be, Bd] = igrfs(latitude, longitude, altitude)

% Fundamental constant.
Rearth_km = 6371.2;

%%% CHECK INPUT VALIDITY %%%
% Convert time to a datenumber if it is a string.
% if ischar(time)
%     time = datenum(time);
% end

% Check that the input coordinates are scalars.
if ~isscalar(latitude) || ~isscalar(longitude) || ~isscalar(altitude)
    error('igrf1:inputNotScalar', ...
        'The input coordinates must be scalars.');
end

%%% SPHERICAL COORDINATE CONVERSION %%%
% Convert the latitude, longitude, and altitude coordinates input into
% spherical coordinates r (radius), theta (inclination angle from +z axis),
% and phi (azimuth angle from +x axis).
% We want cos(theta) and sin(theta) rather than theta itself.
costheta = cos(((pi()/2) - latitude));
sintheta = sin(((pi()/2) - latitude));

% Convert from geodetic coordinates to geocentric coordinates if necessary.
% This method was adapted from igrf11syn, which was a conversion of the
% IGRF subroutine written in FORTRAN.

r = altitude;

% Convert longitude to radians.
phi = longitude; %Conversion in Simulink

%IGRF Coefficient

gh = [-29442	-1501	4797.1	-2445.1	3012.9	-2845.6	1676.7	-641.9	1350.7	-2352.3	-115.3	1225.6	244.9	582	-538.4	907.6	813.7	283.3	120.4	-188.7	-334.9	180.9	70.4	-329.5	-232.6	360.1	47.3	192.4	197	-140.9	-119.3	-157.5	16	4.1	100.2	70	67.7	-20.8	72.7	33.2	-129.9	58.9	-28.9	-66.7	13.2	7.3	-70.9	62.6	81.6	-76.1	-54.1	-6.8	-19.5	51.8	5.7	15	24.4	9.4	3.4	-2.8	-27.4	6.8	-2.2	24.2	8.8	10.1	-16.9	-18.3	-3.2	13.3	-20.6	-14.6	13.4	16.2	11.7	5.7	-15.9	-9.1	-2	2.1	5.4	8.8	-21.6	3.1	10.8	-3.3	11.8	0.7	-6.8	-13.3	-6.9	-0.1	7.8	8.7	1	-9.1	-4	-10.5	8.4	-1.9	-6.3	3.2	0.1	-0.4	0.5	4.6	-0.5	4.4	1.8	-7.9	-0.7	-0.6	2.1	-4.2	2.4	-2.8	-1.8	-1.2	-3.6	-8.7	3.1	-1.5	-0.1	-2.3	2	2	-0.7	-0.8	-1.1	0.6	0.8	-0.7	-0.2	0.2	-2.2	1.7	-1.4	-0.2	-2.5	0.4	-2	3.5	-2.4	-1.9	-0.2	-1.1	0.4	0.4	1.2	1.9	-0.8	-2.2	0.9	0.3	0.1	0.7	0.5	-0.1	-0.3	0.3	-0.4	0.2	0.2	-0.9	-0.9	-0.1	0	0.7	0	-0.9	-0.9	0.4	0.4	0.5	1.6	-0.5	-0.5	1	-1.2	-0.2	-0.1	0.8	0.4	-0.1	-0.1	0.3	0.4	0.1	0.5	0.5	-0.3	-0.4	-0.4	-0.3	-0.8];
gh = transpose(gh);
nmax = sqrt(numel(gh) + 1) - 1;
% We need cos(m*phi) and sin(m*phi) multiple times, so precalculate into a
% vector here:
cosphi = cos((1:nmax)*phi);
sinphi = sin((1:nmax)*phi);

Pmax = (nmax+1)*(nmax+2)/2;

%%% BEGIN MAGNETIC FIELD CALCULATION %%%
% Initialize variables used in for loop below.
Br = 0; Bt = 0; Bp = 0;
 P = zeros(1, Pmax);  P(1) = 1;  P(3) = sintheta;
dP = zeros(1, Pmax); dP(1) = 0; dP(3) = costheta;

% For this initial condition, the first if will result in n = 1, m = 0.
m = 1; n = 0; coefindex = 1;

a_r = (Rearth_km/r)^2;

% Increment through all the n's and m's. gh will be a vector with g
% followed by h for incrementing through n and m except when h would be
% redundant (i.e., when m = 0).
for Pindex = 2:Pmax
    
    % Increment to the next n when m becomes larger than n.
    if n < m
        m = 0;
        n = n + 1;
        a_r = a_r*(Rearth_km/r); % We need (Rearth_km./r)^(n+2)
    end
    
    % Calculate P and dP. They are given recursively according to:
    % 
    % P(0, 0) = 1, P(1, 1) = sin(theta) <- Specified above
    % P(n, n) = sqrt(1 - 1/(2n))*sin(theta)*P(n-1, n-1)
    % P(n, m) = (2n - 1)/sqrt(n^2 - m^2)*cos(theta)*P(n-1, m) -
    %     sqrt(((n-1)^2 - m^2) / (n^2 - m^2)) * P(n-2, m)
    % 
    % dP(0, 0) = 0, dP(1, 1) = cos(theta) <- Specified above
    % dP(n, n) = sqrt(1 - 1/(2n))*(sin(theta)*dP(n-1, n-1) +
    %     cos(theta)*P(n-1, n-1))
    % dP(n, m) = (2n - 1)/sqrt(n^2 - m^2)*(cos(theta)*dP(n-1, m) -
    %     sin(theta)*P(n-1, m)) - sqrt(((n-1)^2 - m^2)/(n^2 - m^2))*
    %     dP(n-2, m)
    if m < n && Pindex ~= 3 % (Pindex=3 is n=1, m=1, initial cond. above)
        last1n = Pindex - n;
        last2n = Pindex - 2*n + 1;
        P(Pindex) = (2*n - 1)/sqrt(n^2 - m^2)*costheta*P(last1n) - ...
            sqrt(((n-1)^2 - m^2) / (n^2 - m^2)) * P(last2n);
        dP(Pindex) = (2*n - 1)/sqrt(n^2 - m^2)*(costheta*dP(last1n) - ...
            sintheta*P(last1n)) - sqrt(((n-1)^2 - m^2) / (n^2 - m^2)) * ...
            dP(last2n);
    elseif Pindex ~= 3
        lastn = Pindex - n - 1;
        P(Pindex) = sqrt(1 - 1/(2*m))*sintheta*P(lastn);
        dP(Pindex) = sqrt(1 - 1/(2*m))*(sintheta*dP(lastn) + ...
            costheta*P(lastn));
    end
    
    % Calculate the magnetic field components as a running sum. Find
    % explicit expressions for these in Global Earth Physics: a Handbook of
    % Physical Constants by Thomas J. Aherns (1995), pg. 49. Link:
    % http://books.google.com/books?id=aqjU_NHyre4C&lpg=PP1&dq=Global%20
    % earth%20physics%3A%20a%20handbook%20of%20physical%20constants&pg=PA49
    % #v=onepage&q&f=false
    % (except equation 6 is missing a required 1/sin(theta) and m; correct
    % equations on page 5 (equations 3a-3c) of:
    % http://hanspeterschaub.info/Papers/UnderGradStudents/
    % MagneticField.pdf)
    if m == 0 % Implies h = 0, so only coefficient in gh is g
        coef = a_r*gh(coefindex); %*cos(0*phi) = 1
        Br = Br + (n+1)*coef*P(Pindex);
        Bt = Bt - coef*dP(Pindex);
        % Bp is 0 for m = 0.
        coefindex = coefindex + 1; % Only need to skip over g this time.
    else
        coef = a_r*(gh(coefindex)*cosphi(m) + gh(coefindex+1)*sinphi(m));
        Br = Br + (n+1)*coef*P(Pindex);
        Bt = Bt - coef*dP(Pindex);
        if sintheta == 0 % Use different formula when dividing by 0.
            Bp = Bp - costheta*a_r*(-gh(coefindex)*sinphi(m) + ...
                gh(coefindex+1)*cosphi(m))*dP(Pindex);
        else
            Bp = Bp - 1/sintheta*a_r*m*(-gh(coefindex)*sinphi(m) + ...
                gh(coefindex+1)*cosphi(m))*P(Pindex);
        end
        coefindex = coefindex + 2; % Skip over g and h this time.
    end
    
    % Increment m.
    m = m + 1;
    
end

% Convert from spherical to (x,y,z) = (North,East,Down).
Bn = -Bt;
Be = Bp;
Bd = -Br;
